simulink model "a2_p3"  (R2019a)
settings: Solver=FixedStepAuto  StartTime=0.0  StopTime=inf  FixedStep=0.01  MaxStep=0.2  RelTol=1e-3  EnableMultiTasking=on
settings Model: EnablePacing=on  PacingRate=3  Creator=YashSeeta  LastModifiedBy=YashSeeta

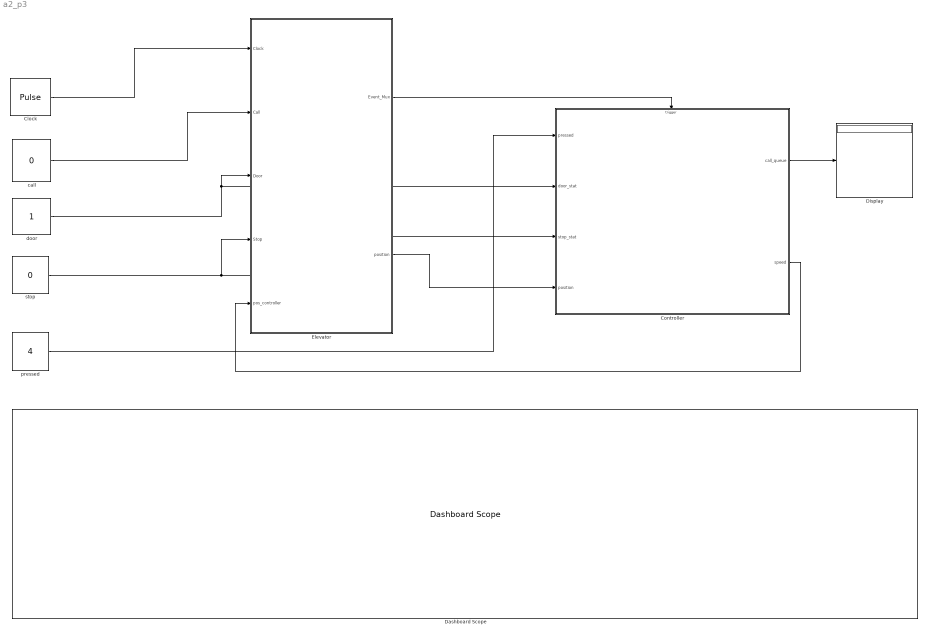
== system a2_p3 ==
  Clock : DiscretePulseGenerator  PulseType=Time based  Period=1  PulseWidth=5
  Controller : Stateflow chart  BlockKeywords=__PRM__SERIALIZED__DATA__:Stateflow Chart,Stateflow Diagram  TreatAsAtomicUnit=on
  Dashboard Scope : DashboardScope  TimeSpan=400  Ymin=0  Ymax=5  ScaleAtStop=off
  Display : Display
  Elevator : Subsystem
  call : Constant  Value=0  OutDataTypeStr=double
  door : Constant  OutDataTypeStr=double
  pressed : Constant  Value=4  OutDataTypeStr=double
  stop : Constant  Value=0  OutDataTypeStr=double
  wires:
  Controller/1(call_queue) -> Display/1
  door/1 -> Elevator/3(Door), Controller/2(door_stat)
  pressed/1 -> Controller/1(pressed)
  Clock/1 -> Elevator/1(Clock)
  call/1 -> Elevator/2(Call)
  Controller/2(speed) -> Elevator/5(pos_controller)
  Elevator/1(Event_Mux) -> Controller/Trigger
  Elevator/2(position) -> Controller/4(position)
  stop/1 -> Elevator/4(Stop), Controller/3(stop_stat)

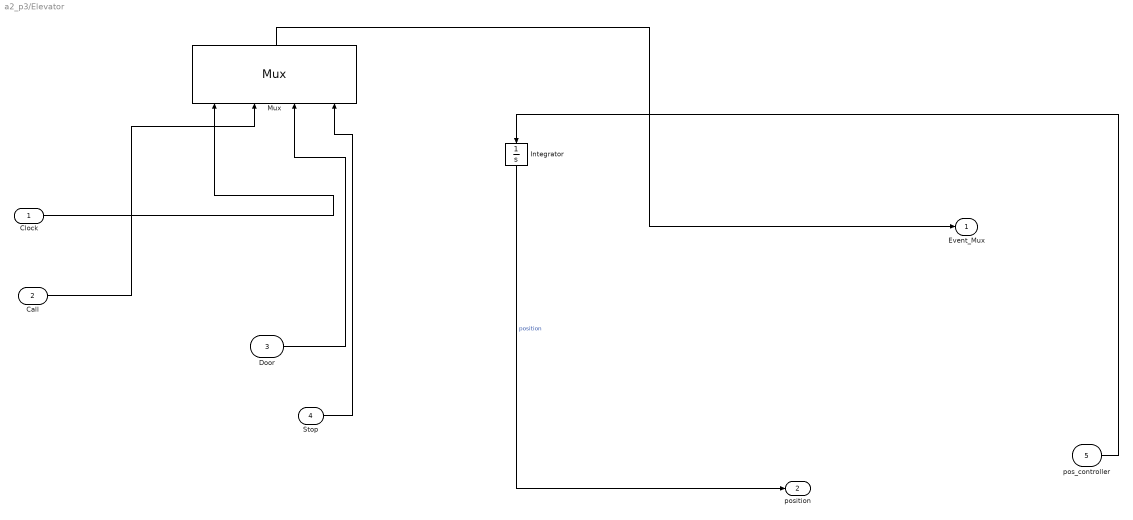
== system a2_p3/Elevator ==
  Clock : Inport
  Call : Inport  Port=2
  Door : Inport  Port=3
  Stop : Inport  Port=4
  pos_controller : Inport  Port=5
  Integrator : Integrator  InitialCondition=1
  Mux : Mux
      settings: DisplayOption=signals
  Event_Mux : Outport
  position : Outport  Port=2
  wires:
  Door/1 -> Mux/3
  Call/1 -> Mux/2
  Mux/1 -> Event_Mux/1
  Integrator/1 -> position/1  "position"
  Stop/1 -> Mux/4
  Clock/1 -> Mux/1
  pos_controller/1 -> Integrator/1

== stateflow chart a2_p3/Controller ==
  settings: executeAtInitialization=1
  state speed = set_speed(position) [function]
    note: % when going down maintain
        | full speed
    note: % when going up maintain
        | full speed
    note: % when going down  and within
        | SLOW_RANGE of goal, slown down
        | the elevator.
    note: % when going up and within
        | SLOW_RANGE of goal, slown down
        | the elevator.
    note: % stop elevator when the position is within the
        | MARGIN range of goal
    (default) -> (junction 75) : {goal = call_queue[0] ;}
    (junction 78) -> (junction 224) [order 2]
    (junction 75) -> (junction 78) [order 1] : [position > goal + MARGIN ]
        | {speed = -MAX_SPEED;}
    (junction 75) -> (junction 105) [order 2] : [position < goal - MARGIN]
        | {speed = MAX_SPEED}
    (junction 105) -> (junction 220) [order 2]
    (junction 78) -> (junction 222) [order 1] : [position - SLOW_RANGE  < goal]
        | {speed = -MAX_SPEED/ 10}
    (junction 75) -> (junction 112) [order 3] : {speed = 0; dq = 1;}
    (junction 105) -> (junction 218) [order 1] : [position + SLOW_RANGE  > goal]
        | {speed = MAX_SPEED/ 10}
  state ButtonControl [parallel]
    settings: executionOrder=1
    state QUEUING
      du:
      on call : nq_floor(pressed);
    (default) -> QUEUING : {ml.try_p3('init');}
  state MovementControl [parallel]
    % input all the button events
    % output speed
    settings: executionOrder=2
    state DEFAULT
      state IDLE
        dq = 0;
      state MOVING
        en : ml.try_p3('close');
        du : speed = set_speed(position);
      state DOORS
        %Doors are opened and after
        %5seconds, they are closed.
      (default) -> IDLE
      IDLE -> MOVING [order 2] : [(call_queue[0] != 0)]
      IDLE -> MOVING [order 1] : call
      DOORS -> IDLE : after(5,sec){ml.try_p3('close')}
      MOVING -> DOORS : [dq]
          | {dq_floor();
          |   ml.try_p3('open');}
    state EMERGENCY
      speed = 0;
      %open doors
      ml.try_p3('open');
      %close doors
      ex: ml.try_p3('close');
    (default) -> DEFAULT
    EMERGENCY -> DEFAULT : stop[!stop_stat]{ml.try_p3('off', 'stop');}
    DEFAULT -> EMERGENCY : stop{ml.try_p3('on', 'stop');}
  state nq_floor(floor_num) [function]
    note: Decision Algorithm : First-come-first-served
        |
        | The call_queue is a FIFO queue
        |
        | 1.Check if the i-th element is 0, assign the floor_num
        |    Turn on the floor light.
        | 2. If not check the queue element by element, untill
        |      above condition is met
    (default) -> (junction 52) : {i = 0;}
    (junction 52) -> (junction 52) [order 2] : [i < numFloor - 1]{i = i + 1}
    (junction 52) -> (junction 55) [order 1] : [call_queue[i] == 0]
        | {call_queue[i] = floor_num;
        |   ml.try_p3('on', pressed);}
    (junction 52) -> (junction 65) [order 3]
  state dq_floor [function]
    note: Removes the first element and turns
        | off the corresponding light
    note: %The "old" copy of the last element is deleted
    note: % Copying the queue elements forward,
        |     the last element is copied as
        |     well, so now we have two copies of the
        |     same call, which will be deleted in the
        |     next step
    (default) -> (junction 117) : {dest = call_queue[0]; i = 0;}
    (junction 119) -> (junction 141) [order 3]
    (junction 119) -> (junction 119) [order 1] : [i < numFloor - 1 & call_queue[i+1] != 0]
        | {
        | call_queue[i] = call_queue[i+1];
        | i = i + 1;
        | }
    (junction 117) -> (junction 119) : {call_queue[i] = 0;ml.try_p3('off',dest)}
    (junction 119) -> (junction 139) [order 2] : [call_queue[i] != 0]{call_queue[i] = 0}
  data: goal temporary double; speed function_output double; position function_input double; floor_num function_input double; i temporary double; i temporary double; call_queue output double size=4; pressed input; door_stat input; stop_stat input; MAX_SPEED constant double =0.2; position input double; speed output double; MARGIN constant double =0.05; dq local double; dest local double; numFloor constant double =4; SLOW_RANGE constant double =0.3
  events: clk input RISING_EDGE_EVENT; call input EITHER_EDGE_EVENT; door_in input EITHER_EDGE_EVENT; stop input EITHER_EDGE_EVENT
